simulink model "HumidityController_2019a"  (R2019a)
settings: Solver=FixedStepAuto  StartTime=0.0  StopTime=inf  RelTol=1e-3  EnableMultiTasking=on
libraries: arduinolib x3, Arduino_Additional_Lib x1, LCDlib x1
settings Model: SimulationMode=external  ExtModeTrigDuration=2  Creator=Shyam lal  LastModifiedBy=Shyam lal
settings OptimizationCC: EnhancedBackFolding=on  PassReuseOutputArgsAs=Individual arguments  MaxStackSize=64  OptimizeBlockOrder=speed  DifferentSizesBufferReuse=on  OptimizationCustomize=off
settings DebuggingCC: ParameterTunabilityLossMsg=error
settings HardwareCC: ProdBitPerInt=16  ProdBitPerPointer=16  ProdBitPerSizeT=16  ProdBitPerPtrDiffT=16  ProdLargestAtomicFloat=None  ProdWordSize=8  ProdHWDeviceType=Atmel->AVR
settings SFSimCC: MATLABDynamicMemAlloc=off
settings RTWCC: SystemTargetFile=ert.tlc  HardwareBoard=Arduino Uno  TLCOptions=-aInlineSetEventsForThisBaseRateFcn=TLC_FALSE -aSuppressMultiTaskScheduler=TLC_FALSE -aRateBasedStepFcn=1  TemplateMakefile=ert_default_tmf  GenerateReport=on  Toolchain=Arduino AVR  BuildConfiguration=Faster Runs  IncludeHyperlinkInReport=on  LaunchReport=on  GenerateTraceInfo=on  GenerateTraceReport=on  GenerateTraceReportSl=on  GenerateTraceReportSf=on  GenerateTraceReportEml=on
settings CodeAppCC: ForceParamTrailComments=on  IgnoreCustomStorageClasses=off  OperatorAnnotations=on  SimulinkDataObjDesc=on  SFDataObjDesc=on  InsertBlockDesc=on
settings ERTTargetCC: SupportContinuousTime=on  SupportVariableSizeSignals=on  ExtModeStaticAllocSize=250

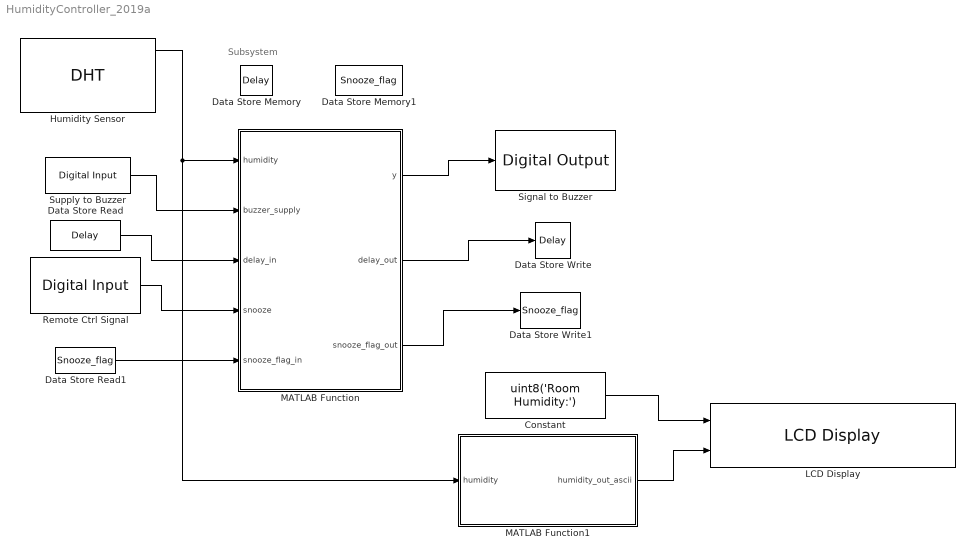
== system HumidityController_2019a ==
  note: Subsystem
  Constant : Constant  Value=uint8('Room Humidity:')
  Data Store Memory : DataStoreMemory  DataStoreName=Delay  ReadBeforeWriteMsg=warning  WriteAfterWriteMsg=warning  WriteAfterReadMsg=warning  InitialValue=150  ShowAdditionalParam=off
  Data Store Memory1 : DataStoreMemory  DataStoreName=Snooze_flag  ReadBeforeWriteMsg=warning  WriteAfterWriteMsg=warning  WriteAfterReadMsg=warning  ShowAdditionalParam=off
  Data Store Read : DataStoreRead  DataStoreName=Delay
  Data Store Read1 : DataStoreRead  DataStoreName=Snooze_flag
  Data Store Write : DataStoreWrite  DataStoreName=Delay
  Data Store Write1 : DataStoreWrite  DataStoreName=Snooze_flag
  "Humidity Sensor " : Arduino_Additional_Lib/DHT  F=off  Pin=5  Tp=11  Ts=0.1
      settings: SourceProductName=Arduino Additional Sensors Library
  LCD Display : LCDlib/LCD Display  pins=[6,7,8,9,10,11]
      settings: SourceProductName=LCD Library
  MATLAB Function : MATLAB Function  TreatAsAtomicUnit=on
  MATLAB Function1 : MATLAB Function  TreatAsAtomicUnit=on
  Remote Ctrl Signal : arduinolib/Digital Input  pinNumber=4  sampleTime=0.1  blockPlatform=arduino
      settings: SourceProductName=Simulink Support Package for Arduino Hardware
  Signal to Buzzer : arduinolib/Digital Output  pinNumber=13  blockPlatform=arduino
  Supply to Buzzer : arduinolib/Digital Input  pinNumber=3  sampleTime=0.1  blockPlatform=arduino
      settings: SourceProductName=Simulink Support Package for Arduino Hardware
  wires:
  "Humidity Sensor "/1 -> MATLAB Function1/1(humidity), MATLAB Function/1(humidity)
  MATLAB Function/1(y) -> Signal to Buzzer/1
  Supply to Buzzer/1 -> MATLAB Function/2(buzzer_supply)
  MATLAB Function1/1(humidity_out_ascii) -> LCD Display/2
  Constant/1 -> LCD Display/1
  Data Store Read/1 -> MATLAB Function/3(delay_in)
  Remote Ctrl Signal/1 -> MATLAB Function/4(snooze)
  MATLAB Function/2(delay_out) -> Data Store Write/1
  Data Store Read1/1 -> MATLAB Function/5(snooze_flag_in)
  MATLAB Function/3(snooze_flag_out) -> Data Store Write1/1

== matlab function HumidityController_2019a/MATLAB Function1 ==
  data: humidity_out_ascii output; humidity input
% Program lcd_switch.m:
% Displays the current humidity of the room to LCD Display 
% by converting the Interger humidity value to ASCII speed value using a switch case.
% Created on Feb 22, 2020 by SHYAM LAL LAKSHMIRAMIYA SRIDHAR

% Input Variables:
% humidity = Integer value of current humidity.

% Output Variables:
% humidity_out_ascii = corresponding humidity value in ASCII format.

function humidity_out_ascii = lcd_switch(humidity)
switch humidity
    case 0
        humidity_out_ascii = [[48],[48]];
    case 1
        humidity_out_ascii = [[48],[49]];
    case 2 
        humidity_out_ascii = [[48],[50]];
    case 3
        humidity_out_ascii = [[48],[51]];
    case 4
        humidity_out_ascii = [[48],[52]];
    case 5
        humidity_out_ascii = [[48],[53]];
    case 6
        humidity_out_ascii = [[48],[54]];
    case 7
        humidity_out_ascii = [[48],[55]];
    case 8
        humidity_out_ascii = [[48],[56]];
    case 9
        humidity_out_ascii = [[48],[57]];
    case 10
        humidity_out_ascii = [[49],[48]];
    case 11 
        humidity_out_ascii = [[49],[49]];
    case 12
        humidity_out_ascii = [[49],[50]];
    case 13
        humidity_out_ascii = [[49],[51]];
    case 14
        humidity_out_ascii = [[49],[52]];
    case 15
        humidity_out_ascii = [[49],[53]];
    case 16
        humidity_out_ascii = [[49],[54]];
    case 17
        humidity_out_ascii = [[49],[55]];
    case 18
        humidity_out_ascii = [[49],[56]];
    case 19
        humidity_out_ascii = [[49],[57]];
    case 20
        humidity_out_ascii = [[50],[48]];
    case 21 
        humidity_out_ascii = [[50],[49]];
    case 22
        humidity_out_ascii = [[50],[50]];
    case 23
        humidity_out_ascii = [[50],[51]];
    case 24
        humidity_out_ascii = [[50],[52]];
    case 25
        humidity_out_ascii = [[50],[53]];
    case 26
        humidity_out_ascii = [[50],[54]];
    case 27
        humidity_out_ascii = [[50],[55]];
    case 28
        humidity_out_ascii = [[50],[56]];
    case 29
        humidity_out_ascii = [[50],[57]];
    case 30
        humidity_out_ascii = [[51],[48]];
    case 31 
        humidity_out_ascii = [[51],[49]];
    case 32
        humidity_out_ascii = [[51],[50]];
    case 33
        humidity_out_ascii = [[51],[51]];
    case 34
        humidity_out_ascii = [[51],[52]];
    case 35
        humidity_out_ascii = [[51],[53]];
    case 36
        humidity_out_ascii = [[51],[54]];
    case 37
        humidity_out_ascii = [[51],[55]];
    case 38
        humidity_out_ascii = [[51],[56]];
    case 39
        humidity_out_ascii = [[51],[57]];
    case 40
        humidity_out_ascii = [[52],[48]];
    case 41 
        humidity_out_ascii = [[52],[49]];
    case 42
        humidity_out_ascii = [[52],[50]];
    case 43
        humidity_out_ascii = [[52],[51]];
    case 44
        humidity_out_ascii = [[52],[52]];
    case 45
        humidity_out_ascii = [[52],[53]];
    case 46
        humidity_out_ascii = [[52],[54]];
    case 47
        humidity_out_ascii = [[52],[55]];
    case 48
        humidity_out_ascii = [[52],[56]];
    case 49
        humidity_out_ascii = [[52],[57]];
    case 50
        humidity_out_ascii = [[53],[48]];
    case 51 
        humidity_out_ascii = [[53],[49]];
    case 52
        humidity_out_ascii = [[53],[50]];
    case 53
        humidity_out_ascii = [[53],[51]];
    case 54
        humidity_out_ascii = [[53],[52]];
    case 55
        humidity_out_ascii = [[53],[53]];
    case 56
        humidity_out_ascii = [[53],[54]];
    case 57
        humidity_out_ascii = [[53],[55]];
    case 58
        humidity_out_ascii = [[53],[56]];
    case 59
        humidity_out_ascii = [[53],[57]];
    case 60
        humidity_out_ascii = [[54],[48]];
    case 61 
        humidity_out_ascii = [[54],[49]];
    case 62
        humidity_out_ascii = [[54],[50]];
    case 63
        humidity_out_ascii = [[54],[51]];
    case 64
        humidity_out_ascii = [[54],[52]];
    case 65
        humidity_out_ascii = [[54],[53]];
    case 66
        humidity_out_ascii = [[54],[54]];
    case 67
        humidity_out_ascii = [[54],[55]];
    case 68
        humidity_out_ascii = [[54],[56]];
    case 69
        humidity_out_ascii = [[54],[57]];
    case 70
        humidity_out_ascii = [[55],[48]];
    case 71 
        humidity_out_ascii = [[55],[49]];
    case 72
        humidity_out_ascii = [[55],[50]];
    case 73
        humidity_out_ascii = [[55],[51]];
    case 74
        humidity_out_ascii = [[55],[52]];
    case 75
        humidity_out_ascii = [[55],[53]];
    case 76
        humidity_out_ascii = [[55],[54]];
    case 77
        humidity_out_ascii = [[55],[55]];
    case 78
        humidity_out_ascii = [[55],[56]];
    case 79
        humidity_out_ascii = [[55],[57]];
    case 80
        humidity_out_ascii = [[56],[48]];
    case 81 
        humidity_out_ascii = [[56],[49]];
    case 82
        humidity_out_ascii = [[56],[50]];
    case 83
        humidity_out_ascii = [[56],[51]];
    case 84
        humidity_out_ascii = [[56],[52]];
    case 85
        humidity_out_ascii = [[56],[53]];
    case 86
        humidity_out_ascii = [[56],[54]];
    case 87
        humidity_out_ascii = [[56],[55]];
    case 88
        humidity_out_ascii = [[56],[56]];
    case 89
        humidity_out_ascii = [[56],[57]];
    case 90
        humidity_out_ascii = [[57],[48]];
    case 91 
        humidity_out_ascii = [[57],[49]];
    case 92
        humidity_out_ascii = [[57],[50]];
    case 93
        humidity_out_ascii = [[57],[51]];
    case 94
        humidity_out_ascii = [[57],[52]];
    case 95
        humidity_out_ascii = [[57],[53]];
    case 96
        humidity_out_ascii = [[57],[54]];
    case 97
        humidity_out_ascii = [[57],[55]];
    case 98
        humidity_out_ascii = [[57],[56]];
    case 99
        humidity_out_ascii = [[57],[57]];
    otherwise
        humidity_out_ascii = [[48],[48]];
end

== matlab function HumidityController_2019a/MATLAB Function ==
  data: humidity input; y output; buzzer_supply input; delay_in input; snooze input; delay_out output; snooze_flag_in input; snooze_flag_out output
function [y, delay_out, snooze_flag_out]  = humidity_controller(humidity, buzzer_supply, delay_in, snooze, snooze_flag_in)

if(humidity<30 || humidity>50) %ideal humidity is 30% to 50%
    ctr=1;
else
    ctr=0;
end
if(~snooze)%snooze==1 normally, without button press
    snooze_flag_out=1;
else
    snooze_flag_out=0;
end
if(snooze_flag_in==0)%snooze button not pressed
    if(ctr==1)
        y=buzzer_supply;
        delay_out=delay_in;
    else
        y=false;
        delay_out=delay_in;
    end  
else %snooze button pressed
    if(delay_in>0)
        y=false;
        delay_out=delay_in-1;
        snooze_flag_out=snooze_flag_in;
    else
        delay_out=150;
        y=false;
        snooze_flag_out=0;
    end
end

end
